simulink model "Formation_Based_Distance"  (R2025a)
settings: Solver=FixedStepAuto  StartTime=0.0  StopTime=10  FixedStep=0.01  RelTol=1e-3
model workspace (MAT data in the model file):
  params : Simulink.Parameter (value not decoded)
values from neighbouring files (symbols this model uses):
  edges = getappdata(0, 'DataEdges')    [DataAnalysis.m]    (also in Data_Analysis.m = graph_params.edges; Trajectory.m = getappdata(0, 'Edges'); consensus_attack.m = [edges_center; edges_circle; edges_diagonal]; data.m = graph_params.edges)
  p10_init = [9; 5; 0]    [data.m]
  p2_init = [10; 0; 0]    [data.m]
  p3_init = [0; 10; 0]    [data.m]
  p4_init = [-10; 0; 0]    [data.m]
  p5_init = [0; -10; 0]    [data.m]
  p6_init = [7; 7; 0]    [data.m]
  p7_init = [-7; 7; 0]    [data.m]
  p8_init = [-7; -7; 0]    [data.m]
  p9_init = [7; -7; 0]    [data.m]
(part 3 of 3)

== matlab function Formation_Based_Distance/Drone 4/MATLAB Function1 ==
  data: p input; v input; pes input; v_star_prev input; v1 input; u output; params parameter Bus: params_bus; v_star output; d_star input; Phi_c output; Phi_a output; gradV_total output
function [u, v_star, Phi_c, Phi_a, gradV_total]  = MATLAB_Function1(p, v, pes, v_star_prev, v1, params, d_star)
    
    graph_params = params.graph_params;
    formation_params = params.formation_params;
    conn_params = params.conn_params;
    avoid_params = params.avoid_params;
    prior_params = params.prior_params;

    
    % Định nghĩa graph_params.edges (9 cạnh)

    n_edges = size(graph_params.edges, 1);
    
    % Chuyển vector p thành mảng 3x5
    pos = reshape(p, 3, graph_params.n_drones);
    vel = reshape(v, 3, graph_params.n_drones);
    pes = reshape(pes, 3, graph_params.n_drones);
    
    % Drone đang xét
    i_drone = 4;

    dt = 0.01;
    
    % =====================================================================
    %  FORMATION CONTROL (Distance-based + Backstepping)
    % =====================================================================
    u_form = zeros(3,1);
    gradV = zeros(3,1);
    
    for e = 1:n_edges
        if graph_params.edges(e,1) == i_drone
            j = graph_params.edges(e,2);
            p_ij = pos(:,j) - pos(:,i_drone);
            v_ij = vel(:,j) - vel(:,i_drone);
            dij = norm(p_ij);
            
            if dij > 1e-6
                e_ij = dij^2 - d_star(e)^2;
                
                % Lực formation (gradient descent)
                u_form = u_form + formation_params.alpha * e_ij * p_ij;
                
                % Gradient V
                gradV = gradV + e_ij * p_ij;
            end
            
        elseif graph_params.edges(e,2) == i_drone
            j = graph_params.edges(e,1);
            p_ij = pos(:,j) - pos(:,i_drone);
            v_ij = vel(:,j) - vel(:,i_drone);
            dij = norm(p_ij);
            
            if dij > 1e-6
                e_ij = dij^2 - d_star(e)^2;
                
                u_form = u_form + formation_params.alpha * e_ij * p_ij;
                gradV = gradV + e_ij * p_ij;
            end
        end
    end
    
    
    
    % =====================================================================
    %  CONNECTIVITY MAINTENANCE
    % =====================================================================
    % Tính ma trận kề sigmoid
    A = zeros(graph_params.n_drones);
    for i = 1:graph_params.n_drones
        for j = i+1:graph_params.n_drones
            d_ij = norm(pos(:,i) - pos(:,j));
            a_ij = 1 / (1 + exp(-conn_params.omega * (conn_params.epsilon - d_ij/conn_params.d_max)));
            A(i,j) = a_ij;
            A(j,i) = a_ij;
        end
    end
    
    % Ma trận Laplace
    D = diag(sum(A,2));
    L = D - A;
    
    Q = conn_params.Q;
    % Tính M = Q'*L*Q
    M = Q' * L * Q;
    lambda2 = min(eig(M));
    
    detM = det(M);
    if detM < 1e-6
        detM = 1e-6;
    end

    Phi_c = 1/(detM^(conn_params.alpha));
    
    % Tính lực giữ liên kết bằng sai phân số
    u_conn = zeros(3, 1);
    eps_fd = 1e-4;
    
    for d = 1:graph_params.dim
        % M tại p + eps
        pos_plus = pos;
        pos_plus(d, i_drone) = pos_plus(d, i_drone) + eps_fd;
        
        A_plus = zeros(graph_params.n_drones);
        for i = 1:graph_params.n_drones
            for j = i+1:graph_params.n_drones
                d_ij = norm(pos_plus(:,i) - pos_plus(:,j));
                a_ij = 1 / (1 + exp(-conn_params.omega * (conn_params.epsilon - d_ij/conn_params.d_max)));
                A_plus(i,j) = a_ij;
                A_plus(j,i) = a_ij;
            end
        end
        D_plus = diag(sum(A_plus,2));
        L_plus = D_plus - A_plus;
        M_plus = Q' * L_plus * Q;
        
        % M tại p - eps
        pos_minus = pos;
        pos_minus(d, i_drone) = pos_minus(d, i_drone) - eps_fd;
        
        A_minus = zeros(graph_params.n_drones);
        for i = 1:graph_params.n_drones
            for j = i+1:graph_params.n_drones
                d_ij = norm(pos_minus(:,i) - pos_minus(:,j));
                a_ij = 1 / (1 + exp(-conn_params.omega * (conn_params.epsilon - d_ij/conn_params.d_max)));
                A_minus(i,j) = a_ij;
                A_minus(j,i) = a_ij;
            end
        end
        D_minus = diag(sum(A_minus,2));
        L_minus = D_minus - A_minus;
        M_minus = Q' * L_minus * Q;
        
        dM_dp = (M_plus - M_minus) / (2*eps_fd);
        
        if rcond(M) > 1e-6
            u_conn(d) = conn_params.alpha * trace(M \ dM_dp) / detM^conn_params.alpha;
        else
            u_conn(d) = 0;
        end
    end
    
    % =====================================================================
    %  OBSTACLE AVOIDANCE
    % =====================================================================
    muy = (1 + avoid_params.d_safe^4) / avoid_params.d_safe^4;
    
    % Tính beta_product
    beta_product = 1;
    for e = 1:n_edges
        i = graph_params.edges(e,1);
        j = graph_params.edges(e,2);
        dij = norm(pos(:,i) - pos(:,j));
        beta_val = beta_slide(dij, avoid_params.d_safe, muy);
        beta_product = beta_product * beta_val;
    end
    
    Phi_a = 1 / (beta_product^avoid_params.alpha);
    dPhi_dbeta = -avoid_params.alpha * beta_product^(-avoid_params.alpha-1);
    
    % Tính lực tránh
    u_avoid = zeros(3, 1);
    eps_deriv = 1e-4;
    
    for j = 1:graph_params.n_drones
        if j == i_drone
            continue;
        end
        
        p_ij = pos(:,i_drone) - pos(:,j);
        dij_ij = norm(p_ij);
        
        if dij_ij > 1e-6
            dd_dp = p_ij;
            
            % Đạo hàm số của beta
            beta_plus = beta_slide(dij_ij + eps_deriv, avoid_params.d_safe, muy);
            beta_minus = beta_slide(dij_ij - eps_deriv, avoid_params.d_safe, muy);
            dbeta_dd = (beta_plus - beta_minus) / (2*eps_deriv);
            
            grad = dPhi_dbeta * dbeta_dd * dd_dp;
            u_avoid = u_avoid - avoid_params.k * grad;
        end
    end

    gradV_total = -prior_params.k_form*u_form - prior_params.k_avoid*u_avoid - prior_params.k_conn*u_conn;

    gradV_total = max(min(gradV_total, 30), -30);

    z3 = [0; 0; (pes(3, i_drone) - pos(3,1))];

    v_star = -formation_params.kd*gradV_total + v1 - prior_params.k_height*z3;

    dv_star = (v_star - v_star_prev) / dt;

    dv_star = max(min(dv_star, 50), -50);
    
    % =====================================================================
    %  TỔNG HỢP
    % =====================================================================
    u = -formation_params.K2 * (vel(:, i_drone) - v_star) + dv_star - gradV_total - z3;
    
end

function beta = beta_slide(dist, d_safe, muy)
    if (dist^2 - d_safe^2) >= 0
        rho = 0;
    else
        rho = 1;
    end
    diff_sq = (dist^2 - d_safe^2)^2;
    beta = (1 - muy * diff_sq / (1 + diff_sq))^rho;
    % Đảm bảo beta không âm
    beta = max(beta, 0);
end

== matlab function Formation_Based_Distance/Drone 1/Subsystem1/Kinematic ==
  data: p_ddot output; u input
function p_ddot = fcn(u)

    p_ddot = u;

end

== matlab function Formation_Based_Distance/Drone 2/MATLAB Function1 ==
  data: p input; v input; pes input; v_star_prev input; v1 input; u output; params parameter Bus: params_bus; v_star output; d_star input; Phi_c output; Phi_a output; gradV_total output
function [u, v_star, Phi_c, Phi_a, gradV_total]  = MATLAB_Function1(p, v, pes, v_star_prev, v1, params, d_star)
    
    graph_params = params.graph_params;
    formation_params = params.formation_params;
    conn_params = params.conn_params;
    avoid_params = params.avoid_params;
    prior_params = params.prior_params;

    
    % Định nghĩa graph_params.edges (9 cạnh)

    n_edges = size(graph_params.edges, 1);
    
    % Chuyển vector p thành mảng 3x5
    pos = reshape(p, 3, graph_params.n_drones);
    vel = reshape(v, 3, graph_params.n_drones);
    pes = reshape(pes, 3, graph_params.n_drones);
    
    % Drone đang xét
    i_drone = 2;

    dt = 0.01;
    
    % =====================================================================
    %  FORMATION CONTROL (Distance-based + Backstepping)
    % =====================================================================
    u_form = zeros(3,1);
    gradV = zeros(3,1);
    
    for e = 1:n_edges
        if graph_params.edges(e,1) == i_drone
            j = graph_params.edges(e,2);
            p_ij = pos(:,j) - pos(:,i_drone);
            v_ij = vel(:,j) - vel(:,i_drone);
            dij = norm(p_ij);
            
            if dij > 1e-6
                e_ij = dij^2 - d_star(e)^2;
                
                % Lực formation (gradient descent)
                u_form = u_form + formation_params.alpha * e_ij * p_ij;
                
                % Gradient V
                gradV = gradV + e_ij * p_ij;
            end
            
        elseif graph_params.edges(e,2) == i_drone
            j = graph_params.edges(e,1);
            p_ij = pos(:,j) - pos(:,i_drone);
            v_ij = vel(:,j) - vel(:,i_drone);
            dij = norm(p_ij);
            
            if dij > 1e-6
                e_ij = dij^2 - d_star(e)^2;
                
                u_form = u_form + formation_params.alpha * e_ij * p_ij;
                gradV = gradV + e_ij * p_ij;
            end
        end
    end
    
    
    
    % =====================================================================
    %  CONNECTIVITY MAINTENANCE
    % =====================================================================
    % Tính ma trận kề sigmoid
    A = zeros(graph_params.n_drones);
    for i = 1:graph_params.n_drones
        for j = i+1:graph_params.n_drones
            d_ij = norm(pos(:,i) - pos(:,j));
            a_ij = 1 / (1 + exp(-conn_params.omega * (conn_params.epsilon - d_ij/conn_params.d_max)));
            A(i,j) = a_ij;
            A(j,i) = a_ij;
        end
    end
    
    % Ma trận Laplace
    D = diag(sum(A,2));
    L = D - A;
    
    Q = conn_params.Q;
    % Tính M = Q'*L*Q
    M = Q' * L * Q;
    lambda2 = min(eig(M));
    
    detM = det(M);
    if detM < 1e-6
        detM = 1e-6;
    end
    Phi_c = 1/(detM)^(conn_params.alpha);
    
    % Tính lực giữ liên kết bằng sai phân số
    u_conn = zeros(3, 1);
    eps_fd = 1e-4;
    
    for d = 1:graph_params.dim
        % M tại p + eps
        pos_plus = pos;
        pos_plus(d, i_drone) = pos_plus(d, i_drone) + eps_fd;
        
        A_plus = zeros(graph_params.n_drones);
        for i = 1:graph_params.n_drones
            for j = i+1:graph_params.n_drones
                d_ij = norm(pos_plus(:,i) - pos_plus(:,j));
                a_ij = 1 / (1 + exp(-conn_params.omega * (conn_params.epsilon - d_ij/conn_params.d_max)));
                A_plus(i,j) = a_ij;
                A_plus(j,i) = a_ij;
            end
        end
        D_plus = diag(sum(A_plus,2));
        L_plus = D_plus - A_plus;
        M_plus = Q' * L_plus * Q;
        
        % M tại p - eps
        pos_minus = pos;
        pos_minus(d, i_drone) = pos_minus(d, i_drone) - eps_fd;
        
        A_minus = zeros(graph_params.n_drones);
        for i = 1:graph_params.n_drones
            for j = i+1:graph_params.n_drones
                d_ij = norm(pos_minus(:,i) - pos_minus(:,j));
                a_ij = 1 / (1 + exp(-conn_params.omega * (conn_params.epsilon - d_ij/conn_params.d_max)));
                A_minus(i,j) = a_ij;
                A_minus(j,i) = a_ij;
            end
        end
        D_minus = diag(sum(A_minus,2));
        L_minus = D_minus - A_minus;
        M_minus = Q' * L_minus * Q;
        
        dM_dp = (M_plus - M_minus) / (2*eps_fd);
        
        if rcond(M) > 1e-6
            u_conn(d) = conn_params.alpha * trace(M \ dM_dp) / detM^conn_params.alpha;
        else
            u_conn(d) = 0;
        end
    end
    
    % =====================================================================
    %  OBSTACLE AVOIDANCE
    % =====================================================================
    muy = (1 + avoid_params.d_safe^4) / avoid_params.d_safe^4;
    
    % Tính beta_product
    beta_product = 1;
    for e = 1:n_edges
        i = graph_params.edges(e,1);
        j = graph_params.edges(e,2);
        dij = norm(pos(:,i) - pos(:,j));
        beta_val = beta_slide(dij, avoid_params.d_safe, muy);
        beta_product = beta_product * beta_val;
    end
    
    Phi_a = 1 / (beta_product^avoid_params.alpha);
    dPhi_dbeta = -avoid_params.alpha * beta_product^(-avoid_params.alpha-1);
    
    % Tính lực tránh
    u_avoid = zeros(3, 1);
    eps_deriv = 1e-4;
    
    for j = 1:graph_params.n_drones
        if j == i_drone
            continue;
        end
        
        p_ij = pos(:,i_drone) - pos(:,j);
        dij_ij = norm(p_ij);
        
        if dij_ij > 1e-6
            dd_dp = p_ij;
            
            % Đạo hàm số của beta
            beta_plus = beta_slide(dij_ij + eps_deriv, avoid_params.d_safe, muy);
            beta_minus = beta_slide(dij_ij - eps_deriv, avoid_params.d_safe, muy);
            dbeta_dd = (beta_plus - beta_minus) / (2*eps_deriv);
            
            grad = dPhi_dbeta * dbeta_dd * dd_dp;
            u_avoid = u_avoid - avoid_params.k * grad;
        end
    end

    gradV_total = -prior_params.k_form*u_form - prior_params.k_avoid*u_avoid - prior_params.k_conn*u_conn;

    gradV_total = max(min(gradV_total, 30), -30);

    z3 = [0; 0; (pes(3, i_drone) - pos(3,1))];

    v_star = -formation_params.kd*gradV_total + v1 - prior_params.k_height*z3;

    dv_star = (v_star - v_star_prev) / dt;

    dv_star = max(min(dv_star, 50), -50);
    
    % =====================================================================
    %  TỔNG HỢP
    % =====================================================================
    u = -formation_params.K2 * (vel(:, i_drone) - v_star) + dv_star - gradV_total - z3;
    
end

function beta = beta_slide(dist, d_safe, muy)
    if (dist^2 - d_safe^2) >= 0
        rho = 0;
    else
        rho = 1;
    end
    diff_sq = (dist^2 - d_safe^2)^2;
    beta = (1 - muy * diff_sq / (1 + diff_sq))^rho;
    % Đảm bảo beta không âm
    beta = max(beta, 0);
end

== matlab function Formation_Based_Distance/Drone 2/Pos Estimation ==
  data: p input; v input; pes input; pes_dot output size=[3, 1]; params parameter Bus: params_bus
function pes_dot = fcn(p, v, pes, params)

    graph_params = params.graph_params;
    estimation_params = params.estimation_params;

    pes_dot = zeros(3,1);
    
    
    i_drone = 2;  % Drone đang xét
    
    % Reshape input
    pos = reshape(p, graph_params.dim, graph_params.n_drones);
    pes = reshape(pes, graph_params.dim, graph_params.n_drones);
    vel = reshape(v, graph_params.dim, graph_params.n_drones);
    
    % Tính toán gradient term
    grad_term = zeros(graph_params.dim, 1);
    
    n_edges = size(graph_params.edges, 1);
    
    for e = 1:n_edges
        if graph_params.edges(e,1) == i_drone
            j = graph_params.edges(e,2);
        else
            j = graph_params.edges(e,1);
        end

        if j == 1
            grad_term = grad_term + ((pos(:, j) - pes(:,i_drone)) - (pos(:, j) - pos(:, i_drone)));
        else
            grad_term = grad_term + (pes(:, j) - pes(:, i_drone) - (pos(:, j) - pos(:, i_drone)));
        end
    end

    
    % Output
    
    pes_dot1 = vel(:, i_drone) + estimation_params.mu*grad_term;
    pes_dot = [pes_dot1(1); pes_dot1(2); pes_dot1(3)];
end
